simulink model "Two_Zone_MVDC_PSolver_R2020b"  (R2020b)
settings: Solver=FixedStepDiscrete  StartTime=0.0  StopTime=30  FixedStep=TsELEC  RelTol=1e-3  EnableMultiTasking=on
InitFcn:
  | TsELEC = 25e-6;
  | Ts = 25e-6;
  | TsTHERMAL = 1e-3;
  | TsCont = TsELEC;
  | Rsnub = 1e4;
undefined symbols (not defined in the file or in its folder): DiscIntNeverNeededParam, ee_sli_rtmsupport, GABDA, GABDB, GBBDA, GBBDB, gcbh, GPMMA, GPPMB, GPPMC, SADA, SADB, SADC, SADD, SBDA, SBDB, SBDC, SCDA, SCDB, SCDC, SCDD, SDDA, SDDB, SDDC, SDDD, SDDE
libraries: fl_lib x138, nesl_utility x69, ee_lib x52, simulink x3, pid_lib x3, eeTransforms x3, sps_avr x2, powerlib_meascontrol x2, slrealtimetgmanagement x1
(part 2 of 4)

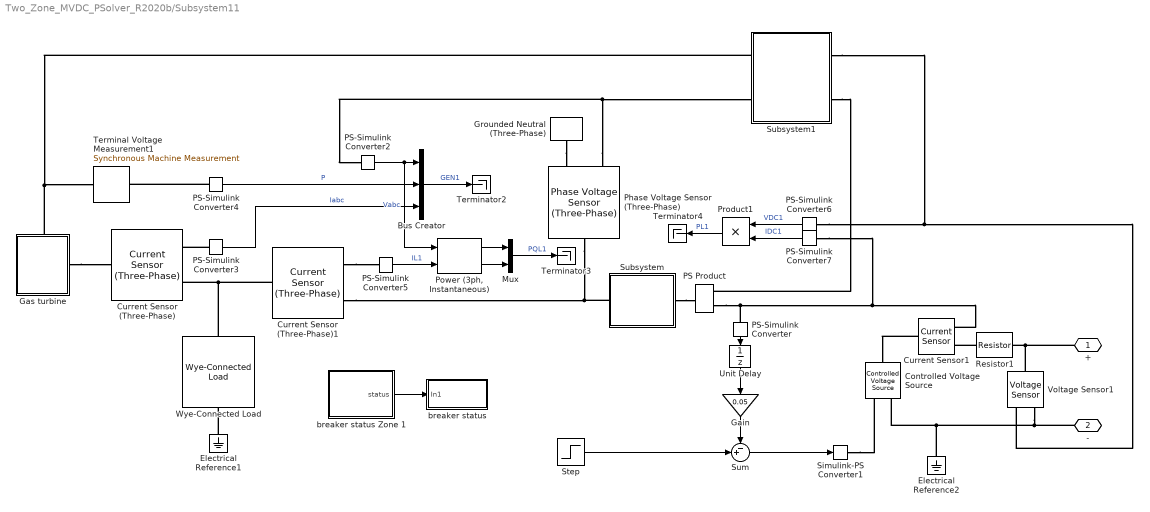
== system Two_Zone_MVDC_PSolver_R2020b/Subsystem11 ==
  Bus Creator : BusCreator  Inputs=3
  Controlled Voltage Source : fl_lib/Electrical/Electrical Sources/Controlled Voltage Source
  Current Sensor (Three-Phase) : ee_lib/Sensors & Transducers/Current Sensor (Three-Phase)
  Current Sensor (Three-Phase)1 : ee_lib/Sensors & Transducers/Current Sensor (Three-Phase)
  Current Sensor1 : fl_lib/Electrical/Electrical Sensors/Current Sensor
  Electrical Reference1 : fl_lib/Electrical/Electrical Elements/Electrical Reference
  Electrical Reference2 : fl_lib/Electrical/Electrical Elements/Electrical Reference
  Gain : Gain  Gain=0.05
  Gas turbine : Subsystem
      settings: PortSchema="{\"entries\":[{\"content\":{\"sides\":[{\"content\":{\"connectorIds\":[]},\"type\":\"ConnectorPlacement.EquallySpacedRectSide\",\"uuid\":\"a1f73c15-13f6-46eb-8342-aad52ebb7cf4\"},{\"content\":{\"connectorIds\":[\"RConn1\"],\"side\":\"RIGHT\"},\"type\":\"ConnectorPlacement.EquallySpacedRectSide\",\"uuid\":\"abeac150-29b8-4860-b513-cf36daae961c\"},{\"content\":{\"connectorIds\":[\"LConn1\"],\"side\":\"TOP\"},\"type\":\"ConnectorPlacement.EquallySpacedRectSide\",\"uuid\":\"5a1fe7e2-6277-4ca3-8dff-8c421d1192c4\"}]},\"type\":\"ConnectorPlacement.EquallySpacedConnector\",\"uuid\":\"d4b4a2cc-ac74-4118-848e-e1a8f51c8633\"}],\"packageUris\":[\"http://schema.mathworks.com/mf0/Connector/19700101\"],\"version\":\"1.0\"}"
  Grounded Neutral (Three-Phase) : ee_lib/Connectors & References/Grounded Neutral (Three-Phase)
      settings: SourceProductBaseCode=PS
  Mux : Mux  Inputs=2
  PS Product : fl_lib/Physical Signals/Functions/PS Product
  PS-Simulink Converter{,2..7} (7 alike) : nesl_utility/PS-Simulink Converter  PhysicalDomain=network_engine_domain  SubClassName=ps_output  LeftPortType=input  RightPortType=output  PseudoPeriodic=off  Frequencies=[]  Unit=inherit  AffineConversion=off
  Phase Voltage Sensor (Three-Phase) : ee_lib/Sensors & Transducers/Phase Voltage Sensor (Three-Phase)
      settings: SourceProductBaseCode=PS
  "Power (3ph, Instantaneous)" : powerlib_meascontrol/Measurements/Power (3ph, Instantaneous)
  Product1 : Product
  Resistor1 : fl_lib/Electrical/Electrical Elements/Resistor  R=1e-5 Ohm  i_specify=off  i_priority=None  i=0 A  i_nominal_specify=off  i_nominal_unit=A  i_nominal_value=1  v_specify=off  v_priority=None  v=0 V  v_nominal_specify=off  v_nominal_unit=V  v_nominal_value=1
  Simulink-PS Converter1 : nesl_utility/Simulink-PS Converter  PhysicalDomain=network_engine_domain  SubClassName=ps_input  LeftPortType=input  RightPortType=output  PseudoPeriodic=off  Frequencies=[]  NoiseDistribution=none  NoiseParameters=[]  Unit=1  AffineConversion=off  FilteringAndDerivatives=provide  SimscapeFilterOrder=1  InputFilterTimeConstant=0.001  UdotUserProvided=0
  Step : Step  Time=12.1  Before=12e3  After=12e3  SampleTime=TsELEC
  Subsystem : Subsystem
  Subsystem1 : Subsystem
  Sum : Sum  Inputs=-+|
  Terminal Voltage Measurement1 : ee_lib/Electromechanical/Synchronous/Synchronous Machine Measurement  output_idx=12
      settings: SourceProductBaseCode=PS  LogSimulationData=on  InternalSimscapePortConfiguration="{\"Bottom\":[],\"Left\":[{\"id\":\"pu_input\",\"label\":\"pu\",\"type\":\"input\"}],\"Right\":[{\"id\":\"pu_output\",\"label\":\"o\",\"type\":\"output\"}],\"Top\":[]}"
  Terminator2 : Terminator
  Terminator3 : Terminator
  Terminator4 : Terminator
  Unit Delay : UnitDelay  SampleTime=TsELEC  HasFrameUpgradeWarning=on
  Voltage Sensor1 : fl_lib/Electrical/Electrical Sensors/Voltage Sensor
  Wye-Connected Load : ee_lib/Passive/RLC Assemblies/Wye-Connected Load  parameterization=2  component_structure=1  component_structure_PQ=1  R=1 Ohm  L=1e-3 H  C=1e-6 F  R_parasitic=1e-6 Ohm  G_parasitic=1e-6 1/Ohm  VRated=13.8e3 V  FRated=60 Hz  P=2.5e6 W  Qpos=1e2 V*A  Qneg=-1e2 V*A  Vmag0=24e3 V  Vang0=0 deg  Freq0=60 Hz  R_parasitic_PQ=1e-6 Ohm  G_parasitic_PQ=1e-6 1/Ohm  IL_specify=on  IL_priority=High  IL=[0, 0, 0] A  IL_nominal_specify=off  IL_nominal_unit=A  IL_nominal_value=1  VC_specify=on  VC_priority=High  VC=[0, 0, 0] V  VC_nominal_specify=off  VC_nominal_unit=V  VC_nominal_value=1
      settings: SourceProductBaseCode=PS
  breaker status : Subsystem
  breaker status Zone 1 : Subsystem
  + : PMIOPort  Side=Right
  - : PMIOPort  Port=2  Side=Right
  wires:
  breaker status Zone 1/1(status) -> breaker status/1(In1)
  Bus Creator/1 -> Terminator2/1  "GEN1"
  PS-Simulink Converter7/1 -> Product1/2  "IDC1"
  "Power (3ph, Instantaneous)"/1 -> Mux/1
  Mux/1 -> Terminator3/1  "PQL1"
  PS-Simulink Converter2/1 -> Bus Creator/1, "Power (3ph, Instantaneous)"/1  "Vabc"
  PS-Simulink Converter5/1 -> "Power (3ph, Instantaneous)"/2  "IL1"
  PS-Simulink Converter4/1 -> Bus Creator/2  "P"
  "Power (3ph, Instantaneous)"/2 -> Mux/2
  Product1/1 -> Terminator4/1  "PL1"
  PS-Simulink Converter6/1 -> Product1/1  "VDC1"
  PS-Simulink Converter3/1 -> Bus Creator/3  "Iabc"
  Step/1 -> Sum/2
  PS-Simulink Converter/1 -> Unit Delay/1
  Sum/1 -> Simulink-PS Converter1/1
  Gain/1 -> Sum/1
  Unit Delay/1 -> Gain/1
  connections:
  Voltage Sensor1/LConn1 -- +/RConn1 -- Resistor1/RConn1
  Subsystem1/RConn1 -- PS-Simulink Converter6/LConn1 -- Voltage Sensor1/RConn1
  Voltage Sensor1/RConn2 -- -/RConn1 -- Electrical Reference2/LConn1 -- Controlled Voltage Source/RConn2
  PS Product/LConn1 -- PS-Simulink Converter7/LConn1 -- Current Sensor1/RConn1 -- PS-Simulink Converter/LConn1
  Phase Voltage Sensor (Three-Phase)/LConn1 -- Current Sensor (Three-Phase)1/RConn2 -- Subsystem/RConn1
  Phase Voltage Sensor (Three-Phase)/RConn1 -- PS-Simulink Converter2/LConn1 -- Subsystem1/LConn2
  Resistor1/LConn1 -- Current Sensor1/RConn2
  Grounded Neutral (Three-Phase)/LConn1 -- Phase Voltage Sensor (Three-Phase)/RConn2
  PS-Simulink Converter3/LConn1 -- Current Sensor (Three-Phase)/RConn1
  Electrical Reference1/LConn1 -- Wye-Connected Load/RConn1
  Current Sensor (Three-Phase)1/LConn1 -- Wye-Connected Load/LConn1 -- Current Sensor (Three-Phase)/RConn2
  Simulink-PS Converter1/RConn1 -- Controlled Voltage Source/RConn1
  Current Sensor (Three-Phase)1/RConn1 -- PS-Simulink Converter5/LConn1
  Current Sensor1/LConn1 -- Controlled Voltage Source/LConn1
  Gas turbine/RConn1 -- Current Sensor (Three-Phase)/LConn1
  PS-Simulink Converter4/LConn1 -- Terminal Voltage Measurement1/RConn1
  Gas turbine/LConn1 -- Subsystem1/LConn1 -- Terminal Voltage Measurement1/LConn1
  Subsystem1/RConn2 -- PS Product/LConn2
  Subsystem/LConn1 -- PS Product/RConn1

== system Two_Zone_MVDC_PSolver_R2020b/Subsystem12 ==
  Inductor2 : fl_lib/Electrical/Electrical Elements/Inductor  l=2.63e-6 H  r=0.16e-3 Ohm  g=0 1/Ohm  i_specify=off  i_priority=None  i=0 A  i_nominal_specify=off  i_nominal_unit=A  i_nominal_value=1  v_specify=off  v_priority=None  v=0 V  v_nominal_specify=off  v_nominal_unit=V  v_nominal_value=1  i_L_specify=off  i_L_priority=High  i_L=0 A  i_L_nominal_specify=off  i_L_nominal_unit=A  i_L_nominal_value=1
  Inductor4 : fl_lib/Electrical/Electrical Elements/Inductor  l=2.63e-6 H  r=0.16e-3 Ohm  g=0 1/Ohm  i_specify=off  i_priority=None  i=0 A  i_nominal_specify=off  i_nominal_unit=A  i_nominal_value=1  v_specify=off  v_priority=None  v=0 V  v_nominal_specify=off  v_nominal_unit=V  v_nominal_value=1  i_L_specify=off  i_L_priority=High  i_L=0 A  i_L_nominal_specify=off  i_L_nominal_unit=A  i_L_nominal_value=1
  Resistor : fl_lib/Electrical/Electrical Elements/Resistor  R=Rsnub Ohm  i_specify=off  i_priority=None  i=0 A  i_nominal_specify=off  i_nominal_unit=A  i_nominal_value=1  v_specify=off  v_priority=None  v=0 V  v_nominal_specify=off  v_nominal_unit=V  v_nominal_value=1
  Resistor1 : fl_lib/Electrical/Electrical Elements/Resistor  R=Rsnub Ohm  i_specify=off  i_priority=None  i=0 A  i_nominal_specify=off  i_nominal_unit=A  i_nominal_value=1  v_specify=off  v_priority=None  v=0 V  v_nominal_specify=off  v_nominal_unit=V  v_nominal_value=1
  "+ " : PMIOPort  Side=Left
  + : PMIOPort  Port=2  Side=Right
  - : PMIOPort  Port=3  Side=Left
  "- " : PMIOPort  Port=4  Side=Right
  connections:
  Inductor2/LConn1 -- "+ "/RConn1 -- Resistor/LConn1
  Inductor4/LConn1 -- -/RConn1 -- Resistor/RConn1
  Inductor2/RConn1 -- Resistor1/LConn1 -- +/RConn1
  Inductor4/RConn1 -- Resistor1/RConn1 -- "- "/RConn1

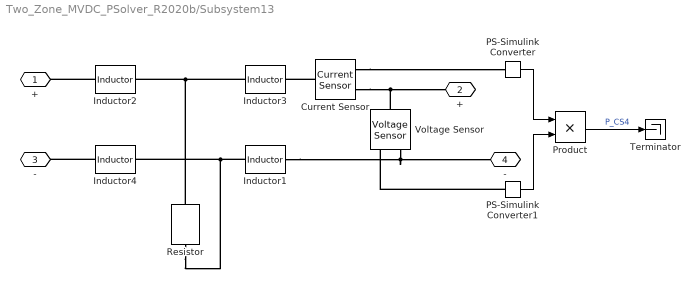
== system Two_Zone_MVDC_PSolver_R2020b/Subsystem13 ==
  Current Sensor : fl_lib/Electrical/Electrical Sensors/Current Sensor
  Inductor{1..4} (4 alike) : fl_lib/Electrical/Electrical Elements/Inductor  l=5e-6/2 H  r=0.2e-3/2 Ohm  g=0 1/Ohm  i_specify=off  i_priority=None  i=0 A  i_nominal_specify=off  i_nominal_unit=A  i_nominal_value=1  v_specify=off  v_priority=None  v=0 V  v_nominal_specify=off  v_nominal_unit=V  v_nominal_value=1  i_L_specify=off  i_L_priority=High  i_L=0 A  i_L_nominal_specify=off  i_L_nominal_unit=A  i_L_nominal_value=1
  PS-Simulink Converter : nesl_utility/PS-Simulink Converter  PhysicalDomain=network_engine_domain  SubClassName=ps_output  LeftPortType=input  RightPortType=output  PseudoPeriodic=off  Frequencies=[]  Unit=inherit  AffineConversion=off
  PS-Simulink Converter1 : nesl_utility/PS-Simulink Converter  PhysicalDomain=network_engine_domain  SubClassName=ps_output  LeftPortType=input  RightPortType=output  PseudoPeriodic=off  Frequencies=[]  Unit=inherit  AffineConversion=off
  Product : Product
  Resistor : fl_lib/Electrical/Electrical Elements/Resistor  R=Rsnub Ohm  i_specify=off  i_priority=None  i=0 A  i_nominal_specify=off  i_nominal_unit=A  i_nominal_value=1  v_specify=off  v_priority=None  v=0 V  v_nominal_specify=off  v_nominal_unit=V  v_nominal_value=1
  Terminator : Terminator
  Voltage Sensor : fl_lib/Electrical/Electrical Sensors/Voltage Sensor
  "+ " : PMIOPort  Side=Left
  + : PMIOPort  Port=2  Side=Right
  - : PMIOPort  Port=3  Side=Left
  "- " : PMIOPort  Port=4  Side=Right
  wires:
  Product/1 -> Terminator/1  "P_CS4"
  PS-Simulink Converter/1 -> Product/1
  PS-Simulink Converter1/1 -> Product/2
  connections:
  Inductor3/LConn1 -- Resistor/LConn1 -- Inductor2/RConn1
  Inductor1/LConn1 -- Resistor/RConn1 -- Inductor4/RConn1
  Current Sensor/LConn1 -- Inductor3/RConn1
  Current Sensor/RConn2 -- Voltage Sensor/LConn1 -- +/RConn1
  Inductor1/RConn1 -- Voltage Sensor/RConn2 -- "- "/RConn1
  Current Sensor/RConn1 -- PS-Simulink Converter/LConn1
  PS-Simulink Converter1/LConn1 -- Voltage Sensor/RConn1
  Inductor2/LConn1 -- "+ "/RConn1
  Inductor4/LConn1 -- -/RConn1

== system Two_Zone_MVDC_PSolver_R2020b/Subsystem14 ==
  Inductor1 : fl_lib/Electrical/Electrical Elements/Inductor  l=5.32e-6 H  r=0.32e-3 Ohm  g=0 1/Ohm  i_specify=off  i_priority=None  i=0 A  i_nominal_specify=off  i_nominal_unit=A  i_nominal_value=1  v_specify=off  v_priority=None  v=0 V  v_nominal_specify=off  v_nominal_unit=V  v_nominal_value=1  i_L_specify=off  i_L_priority=High  i_L=0 A  i_L_nominal_specify=off  i_L_nominal_unit=A  i_L_nominal_value=1
  Inductor2 : fl_lib/Electrical/Electrical Elements/Inductor  l=5.32e-6 H  r=0.32e-3 Ohm  g=0 1/Ohm  i_specify=off  i_priority=None  i=0 A  i_nominal_specify=off  i_nominal_unit=A  i_nominal_value=1  v_specify=off  v_priority=None  v=0 V  v_nominal_specify=off  v_nominal_unit=V  v_nominal_value=1  i_L_specify=off  i_L_priority=High  i_L=0 A  i_L_nominal_specify=off  i_L_nominal_unit=A  i_L_nominal_value=1
  Resistor : fl_lib/Electrical/Electrical Elements/Resistor  R=Rsnub Ohm  i_specify=off  i_priority=None  i=0 A  i_nominal_specify=off  i_nominal_unit=A  i_nominal_value=1  v_specify=off  v_priority=None  v=0 V  v_nominal_specify=off  v_nominal_unit=V  v_nominal_value=1
  "+ " : PMIOPort  Side=Left
  + : PMIOPort  Port=2  Side=Right
  - : PMIOPort  Port=3  Side=Left
  "- " : PMIOPort  Port=4  Side=Right
  connections:
  Inductor1/LConn1 -- Resistor/RConn1 -- -/RConn1
  Inductor2/LConn1 -- Resistor/LConn1 -- "+ "/RConn1
  Inductor2/RConn1 -- +/RConn1
  Inductor1/RConn1 -- "- "/RConn1

== system Two_Zone_MVDC_PSolver_R2020b/Subsystem15 ==
  Inductor1 : fl_lib/Electrical/Electrical Elements/Inductor  l=5.32e-6 H  r=0.32e-3 Ohm  g=0 1/Ohm  i_specify=off  i_priority=None  i=0 A  i_nominal_specify=off  i_nominal_unit=A  i_nominal_value=1  v_specify=off  v_priority=None  v=0 V  v_nominal_specify=off  v_nominal_unit=V  v_nominal_value=1  i_L_specify=off  i_L_priority=High  i_L=0 A  i_L_nominal_specify=off  i_L_nominal_unit=A  i_L_nominal_value=1
  Inductor2 : fl_lib/Electrical/Electrical Elements/Inductor  l=5.32e-6 H  r=0.32e-3 Ohm  g=0 1/Ohm  i_specify=off  i_priority=None  i=0 A  i_nominal_specify=off  i_nominal_unit=A  i_nominal_value=1  v_specify=off  v_priority=None  v=0 V  v_nominal_specify=off  v_nominal_unit=V  v_nominal_value=1  i_L_specify=off  i_L_priority=High  i_L=0 A  i_L_nominal_specify=off  i_L_nominal_unit=A  i_L_nominal_value=1
  Resistor : fl_lib/Electrical/Electrical Elements/Resistor  R=Rsnub Ohm  i_specify=off  i_priority=None  i=0 A  i_nominal_specify=off  i_nominal_unit=A  i_nominal_value=1  v_specify=off  v_priority=None  v=0 V  v_nominal_specify=off  v_nominal_unit=V  v_nominal_value=1
  Resistor1 : fl_lib/Electrical/Electrical Elements/Resistor  R=Rsnub Ohm  i_specify=off  i_priority=None  i=0 A  i_nominal_specify=off  i_nominal_unit=A  i_nominal_value=1  v_specify=off  v_priority=None  v=0 V  v_nominal_specify=off  v_nominal_unit=V  v_nominal_value=1
  "+ " : PMIOPort  Side=Left
  + : PMIOPort  Port=2  Side=Right
  - : PMIOPort  Port=3  Side=Left
  "- " : PMIOPort  Port=4  Side=Right
  connections:
  Inductor1/RConn1 -- Resistor1/LConn1 -- "- "/RConn1
  Inductor2/RConn1 -- Resistor1/RConn1 -- +/RConn1
  Inductor2/LConn1 -- Resistor/LConn1 -- "+ "/RConn1
  Inductor1/LConn1 -- Resistor/RConn1 -- -/RConn1

== system Two_Zone_MVDC_PSolver_R2020b/Subsystem16 ==
  Inductor1 : fl_lib/Electrical/Electrical Elements/Inductor  l=5.32e-6 H  r=0.32e-3 Ohm  g=0 1/Ohm  i_specify=off  i_priority=None  i=0 A  i_nominal_specify=off  i_nominal_unit=A  i_nominal_value=1  v_specify=off  v_priority=None  v=0 V  v_nominal_specify=off  v_nominal_unit=V  v_nominal_value=1  i_L_specify=off  i_L_priority=High  i_L=0 A  i_L_nominal_specify=off  i_L_nominal_unit=A  i_L_nominal_value=1
  Inductor2 : fl_lib/Electrical/Electrical Elements/Inductor  l=5.32e-6 H  r=0.32e-3 Ohm  g=0 1/Ohm  i_specify=off  i_priority=None  i=0 A  i_nominal_specify=off  i_nominal_unit=A  i_nominal_value=1  v_specify=off  v_priority=None  v=0 V  v_nominal_specify=off  v_nominal_unit=V  v_nominal_value=1  i_L_specify=off  i_L_priority=High  i_L=0 A  i_L_nominal_specify=off  i_L_nominal_unit=A  i_L_nominal_value=1
  Resistor : fl_lib/Electrical/Electrical Elements/Resistor  R=Rsnub Ohm  i_specify=off  i_priority=None  i=0 A  i_nominal_specify=off  i_nominal_unit=A  i_nominal_value=1  v_specify=off  v_priority=None  v=0 V  v_nominal_specify=off  v_nominal_unit=V  v_nominal_value=1
  Resistor1 : fl_lib/Electrical/Electrical Elements/Resistor  R=Rsnub Ohm  i_specify=off  i_priority=None  i=0 A  i_nominal_specify=off  i_nominal_unit=A  i_nominal_value=1  v_specify=off  v_priority=None  v=0 V  v_nominal_specify=off  v_nominal_unit=V  v_nominal_value=1
  "+ " : PMIOPort  Side=Left
  + : PMIOPort  Port=2  Side=Right
  - : PMIOPort  Port=3  Side=Left
  "- " : PMIOPort  Port=4  Side=Right
  connections:
  Inductor1/LConn1 -- Resistor/RConn1 -- -/RConn1
  Inductor2/LConn1 -- Resistor/LConn1 -- "+ "/RConn1
  Inductor2/RConn1 -- Resistor1/RConn1 -- +/RConn1
  Inductor1/RConn1 -- Resistor1/LConn1 -- "- "/RConn1

== system Two_Zone_MVDC_PSolver_R2020b/Subsystem2 ==
  Current Sensor : fl_lib/Electrical/Electrical Sensors/Current Sensor
  Inductor1 : fl_lib/Electrical/Electrical Elements/Inductor  l=5e-6 H  r=0.2e-3 Ohm  g=0 1/Ohm  i_specify=off  i_priority=None  i=0 A  i_nominal_specify=off  i_nominal_unit=A  i_nominal_value=1  v_specify=off  v_priority=None  v=0 V  v_nominal_specify=off  v_nominal_unit=V  v_nominal_value=1  i_L_specify=off  i_L_priority=High  i_L=0 A  i_L_nominal_specify=off  i_L_nominal_unit=A  i_L_nominal_value=1
  Inductor3 : fl_lib/Electrical/Electrical Elements/Inductor  l=5e-6 H  r=0.2e-3 Ohm  g=0 1/Ohm  i_specify=off  i_priority=None  i=0 A  i_nominal_specify=off  i_nominal_unit=A  i_nominal_value=1  v_specify=off  v_priority=None  v=0 V  v_nominal_specify=off  v_nominal_unit=V  v_nominal_value=1  i_L_specify=off  i_L_priority=High  i_L=0 A  i_L_nominal_specify=off  i_L_nominal_unit=A  i_L_nominal_value=1
  PS-Simulink Converter : nesl_utility/PS-Simulink Converter  PhysicalDomain=network_engine_domain  SubClassName=ps_output  LeftPortType=input  RightPortType=output  PseudoPeriodic=off  Frequencies=[]  Unit=inherit  AffineConversion=off
  PS-Simulink Converter1 : nesl_utility/PS-Simulink Converter  PhysicalDomain=network_engine_domain  SubClassName=ps_output  LeftPortType=input  RightPortType=output  PseudoPeriodic=off  Frequencies=[]  Unit=inherit  AffineConversion=off
  Product : Product
  Resistor : fl_lib/Electrical/Electrical Elements/Resistor  R=Rsnub Ohm  i_specify=off  i_priority=None  i=0 A  i_nominal_specify=off  i_nominal_unit=A  i_nominal_value=1  v_specify=off  v_priority=None  v=0 V  v_nominal_specify=off  v_nominal_unit=V  v_nominal_value=1
  Resistor1 : fl_lib/Electrical/Electrical Elements/Resistor  R=Rsnub Ohm  i_specify=off  i_priority=None  i=0 A  i_nominal_specify=off  i_nominal_unit=A  i_nominal_value=1  v_specify=off  v_priority=None  v=0 V  v_nominal_specify=off  v_nominal_unit=V  v_nominal_value=1
  Terminator : Terminator
  Voltage Sensor : fl_lib/Electrical/Electrical Sensors/Voltage Sensor
  "+ " : PMIOPort  Side=Left
  + : PMIOPort  Port=2  Side=Right
  - : PMIOPort  Port=3  Side=Left
  "- " : PMIOPort  Port=4  Side=Right
  wires:
  Product/1 -> Terminator/1  "P_CS8"
  PS-Simulink Converter/1 -> Product/1
  PS-Simulink Converter1/1 -> Product/2
  connections:
  Inductor1/LConn1 -- Resistor/RConn1 -- -/RConn1
  Inductor3/LConn1 -- Resistor/LConn1 -- "+ "/RConn1
  Current Sensor/LConn1 -- Resistor1/LConn1 -- Inductor3/RConn1
  Current Sensor/RConn2 -- Voltage Sensor/LConn1 -- +/RConn1
  Inductor1/RConn1 -- Resistor1/RConn1 -- Voltage Sensor/RConn2 -- "- "/RConn1
  Voltage Sensor/RConn1 -- PS-Simulink Converter1/LConn1
  Current Sensor/RConn1 -- PS-Simulink Converter/LConn1

== system Two_Zone_MVDC_PSolver_R2020b/Subsystem3 ==
  Capacitor2 : fl_lib/Electrical/Electrical Elements/Capacitor  c=2e-3 F  r=0 Ohm  g=0 1/Ohm  i_specify=off  i_priority=None  i=0 A  i_nominal_specify=off  i_nominal_unit=A  i_nominal_value=1  v_specify=on  v_priority=None  v=12e3 V  v_nominal_specify=off  v_nominal_unit=V  v_nominal_value=1  vc_specify=on  vc_priority=High  vc=12e3 V  vc_nominal_specify=off  vc_nominal_unit=V  vc_nominal_value=1
  Control : Subsystem
  Current Sensor : fl_lib/Electrical/Electrical Sensors/Current Sensor
  Inverter and PMSM : Subsystem  VariantControl=(sim)
  PS Product : fl_lib/Physical Signals/Functions/PS Product
  PS-Simulink Converter : nesl_utility/PS-Simulink Converter  PhysicalDomain=network_engine_domain  SubClassName=ps_output  LeftPortType=input  RightPortType=output  PseudoPeriodic=off  Frequencies=[]  Unit=inherit  AffineConversion=off
  Speed Reference : Subsystem
  Terminator : Terminator
  Voltage Sensor : fl_lib/Electrical/Electrical Sensors/Voltage Sensor
  + : PMIOPort  Side=Left
  - : PMIOPort  Port=2  Side=Left
  wires:
  PS-Simulink Converter/1 -> Terminator/1  "PDC_motor"
  Control/1(duty_cycle) -> Inverter and PMSM/1(duty_cycle)
  connections:
  PS Product/RConn1 -- PS-Simulink Converter/LConn1
  Voltage Sensor/RConn1 -- PS Product/LConn2
  PS Product/LConn1 -- Current Sensor/RConn1
  Current Sensor/LConn1 -- +/RConn1
  -/RConn1 -- Capacitor2/RConn1 -- Inverter and PMSM/LConn2 -- Voltage Sensor/RConn2
  Capacitor2/LConn1 -- Voltage Sensor/LConn1 -- Current Sensor/RConn2 -- Inverter and PMSM/LConn1

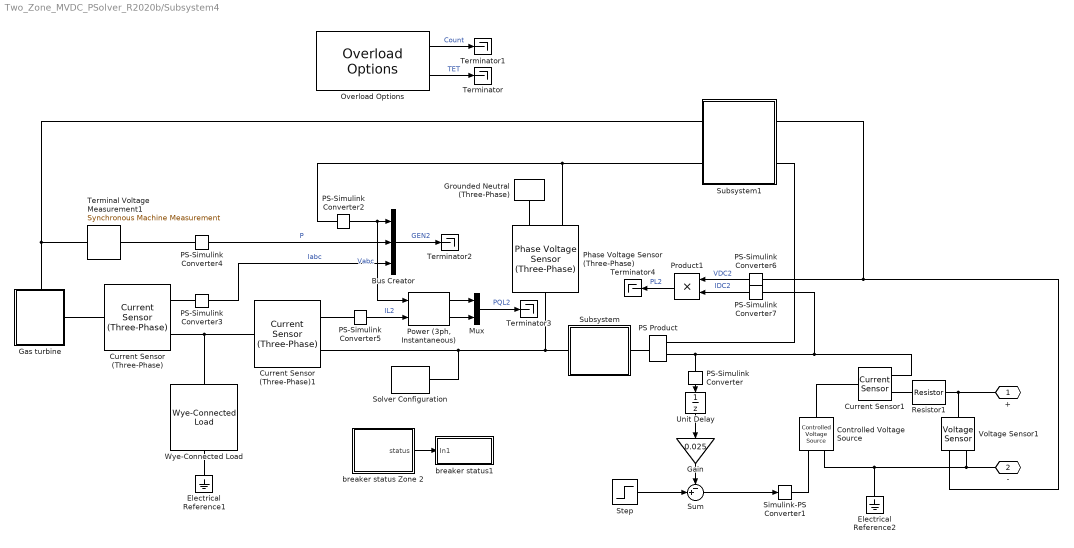
== system Two_Zone_MVDC_PSolver_R2020b/Subsystem4 ==
  Bus Creator : BusCreator  Inputs=3
  Controlled Voltage Source : fl_lib/Electrical/Electrical Sources/Controlled Voltage Source
  Current Sensor (Three-Phase) : ee_lib/Sensors & Transducers/Current Sensor (Three-Phase)
  Current Sensor (Three-Phase)1 : ee_lib/Sensors & Transducers/Current Sensor (Three-Phase)
  Current Sensor1 : fl_lib/Electrical/Electrical Sensors/Current Sensor
  Electrical Reference1 : fl_lib/Electrical/Electrical Elements/Electrical Reference
  Electrical Reference2 : fl_lib/Electrical/Electrical Elements/Electrical Reference
  Gain : Gain  Gain=0.025
  Gas turbine : Subsystem
      settings: PortSchema="{\"entries\":[{\"content\":{\"sides\":[{\"content\":{\"connectorIds\":[]},\"type\":\"ConnectorPlacement.EquallySpacedRectSide\",\"uuid\":\"a1f73c15-13f6-46eb-8342-aad52ebb7cf4\"},{\"content\":{\"connectorIds\":[\"RConn1\"],\"side\":\"RIGHT\"},\"type\":\"ConnectorPlacement.EquallySpacedRectSide\",\"uuid\":\"abeac150-29b8-4860-b513-cf36daae961c\"},{\"content\":{\"connectorIds\":[\"LConn1\"],\"side\":\"TOP\"},\"type\":\"ConnectorPlacement.EquallySpacedRectSide\",\"uuid\":\"5a1fe7e2-6277-4ca3-8dff-8c421d1192c4\"}]},\"type\":\"ConnectorPlacement.EquallySpacedConnector\",\"uuid\":\"d4b4a2cc-ac74-4118-848e-e1a8f51c8633\"}],\"packageUris\":[\"http://schema.mathworks.com/mf0/Connector/19700101\"],\"version\":\"1.0\"}"
  Grounded Neutral (Three-Phase) : ee_lib/Connectors & References/Grounded Neutral (Three-Phase)
      settings: SourceProductBaseCode=PS
  Mux : Mux  Inputs=2
  Overload Options : slrealtimetgmanagement/Overload Options  startupDur=1  startupDurSrc=Tunable Parameter  maxOverload=1000  maxOverloadSrc=Tunable Parameter  TETFlag=on
      settings: SourceProductBaseCode=XP
  PS Product : fl_lib/Physical Signals/Functions/PS Product
  PS-Simulink Converter{,2..7} (7 alike) : nesl_utility/PS-Simulink Converter  PhysicalDomain=network_engine_domain  SubClassName=ps_output  LeftPortType=input  RightPortType=output  PseudoPeriodic=off  Frequencies=[]  Unit=inherit  AffineConversion=off
  Phase Voltage Sensor (Three-Phase) : ee_lib/Sensors & Transducers/Phase Voltage Sensor (Three-Phase)
      settings: SourceProductBaseCode=PS
  "Power (3ph, Instantaneous)" : powerlib_meascontrol/Measurements/Power (3ph, Instantaneous)
  Product1 : Product
  Resistor1 : fl_lib/Electrical/Electrical Elements/Resistor  R=1e-5 Ohm  i_specify=off  i_priority=None  i=0 A  i_nominal_specify=off  i_nominal_unit=A  i_nominal_value=1  v_specify=off  v_priority=None  v=0 V  v_nominal_specify=off  v_nominal_unit=V  v_nominal_value=1
  Simulink-PS Converter1 : nesl_utility/Simulink-PS Converter  PhysicalDomain=network_engine_domain  SubClassName=ps_input  LeftPortType=input  RightPortType=output  PseudoPeriodic=off  Frequencies=[]  NoiseDistribution=none  NoiseParameters=[]  Unit=1  AffineConversion=off  FilteringAndDerivatives=provide  SimscapeFilterOrder=1  InputFilterTimeConstant=0.001  UdotUserProvided=0
  Solver Configuration : nesl_utility/Solver Configuration  PhysicalDomain=network_engine_domain  SubClassName=solver  LeftPortType=input  RightPortType=generic  Tones=[]  Harmonics=[]  SimulateNoise=off  Profile=off  UseLocalSampling=off  EnableSwitchedLinearOptims=on  FrequencyDomain=off  UseCCode=off  RelTol=0.001  AbsTol=1e-06  MinStep=1e-09  ToWorkspace=off  RevertToSquareIcSolve=off  NumHomotopyIterations=100  PhasorMode=off  PhasorModeNumHarmonics=1  DoDC=off  ResidualTolerance=1e-09  UseLocalSolver=on  LocalSolverChoice=NE_PARTITIONING_ADVANCER  LocalSolverSampleTime=TsELEC  DoFixedCost=on  MaxNonlinIter=1  MaxModeIter=2  ComputeImpulses=off  ImpulseIterations=1  LinearAlgebra=auto  EquationFormulation=NE_TIME_EF  DelaysMemoryBudget=1024  AutomaticFiltering=on  FilteringTimeConstant=0.001  PartitionStorageMethod=AS_NEEDED  PartitionMemoryBudget=1024  PartitionMethod=FAST
  Step : Step  Time=12.1  Before=12e3  After=12e3  SampleTime=TsELEC
  Subsystem : Subsystem
  Subsystem1 : Subsystem
  Sum : Sum  Inputs=-+|
  Terminal Voltage Measurement1 : ee_lib/Electromechanical/Synchronous/Synchronous Machine Measurement  output_idx=12
      settings: SourceProductBaseCode=PS  LogSimulationData=on  InternalSimscapePortConfiguration="{\"Bottom\":[],\"Left\":[{\"id\":\"pu_input\",\"label\":\"pu\",\"type\":\"input\"}],\"Right\":[{\"id\":\"pu_output\",\"label\":\"o\",\"type\":\"output\"}],\"Top\":[]}"
  Terminator{,1..4} (5 alike) : Terminator
  Unit Delay : UnitDelay  SampleTime=TsELEC  HasFrameUpgradeWarning=on
  Voltage Sensor1 : fl_lib/Electrical/Electrical Sensors/Voltage Sensor
  Wye-Connected Load : ee_lib/Passive/RLC Assemblies/Wye-Connected Load  parameterization=2  component_structure=1  component_structure_PQ=1  R=1 Ohm  L=1e-3 H  C=1e-6 F  R_parasitic=1e-6 Ohm  G_parasitic=1e-6 1/Ohm  VRated=13.8e3 V  FRated=60 Hz  P=2.5e6 W  Qpos=1e2 V*A  Qneg=-1e2 V*A  Vmag0=24e3 V  Vang0=0 deg  Freq0=60 Hz  R_parasitic_PQ=1e-6 Ohm  G_parasitic_PQ=1e-6 1/Ohm  IL_specify=on  IL_priority=High  IL=[0, 0, 0] A  IL_nominal_specify=off  IL_nominal_unit=A  IL_nominal_value=1  VC_specify=on  VC_priority=High  VC=[0, 0, 0] V  VC_nominal_specify=off  VC_nominal_unit=V  VC_nominal_value=1
      settings: SourceProductBaseCode=PS
  breaker status Zone 2 : Subsystem
  breaker status1 : Subsystem
  + : PMIOPort  Side=Right
  - : PMIOPort  Port=2  Side=Right
  wires:
  breaker status Zone 2/1(status) -> breaker status1/1(In1)
  PS-Simulink Converter6/1 -> Product1/1  "VDC2"
  Product1/1 -> Terminator4/1  "PL2"
  Bus Creator/1 -> Terminator2/1  "GEN2"
  PS-Simulink Converter5/1 -> "Power (3ph, Instantaneous)"/2  "IL2"
  PS-Simulink Converter3/1 -> Bus Creator/3  "Iabc"
  "Power (3ph, Instantaneous)"/1 -> Mux/1
  Mux/1 -> Terminator3/1  "PQL2"
  PS-Simulink Converter2/1 -> Bus Creator/1, "Power (3ph, Instantaneous)"/1  "Vabc"
  PS-Simulink Converter7/1 -> Product1/2  "IDC2"
  "Power (3ph, Instantaneous)"/2 -> Mux/2
  PS-Simulink Converter4/1 -> Bus Creator/2  "P"
  Gain/1 -> Sum/1
  Sum/1 -> Simulink-PS Converter1/1
  Unit Delay/1 -> Gain/1
  Step/1 -> Sum/2
  PS-Simulink Converter/1 -> Unit Delay/1
  Overload Options/2 -> Terminator/1  "TET"
  Overload Options/1 -> Terminator1/1  "Count"
  connections:
  Controlled Voltage Source/RConn2 -- -/RConn1 -- Voltage Sensor1/RConn2 -- Electrical Reference2/LConn1
  Voltage Sensor1/LConn1 -- +/RConn1 -- Resistor1/RConn1
  PS Product/LConn1 -- PS-Simulink Converter/LConn1 -- PS-Simulink Converter7/LConn1 -- Current Sensor1/RConn1
  Phase Voltage Sensor (Three-Phase)/RConn1 -- PS-Simulink Converter2/LConn1 -- Subsystem1/LConn2
  Current Sensor (Three-Phase)1/LConn1 -- Wye-Connected Load/LConn1 -- Current Sensor (Three-Phase)/RConn2
  Subsystem1/RConn1 -- PS-Simulink Converter6/LConn1 -- Voltage Sensor1/RConn1
  Terminal Voltage Measurement1/LConn1 -- Subsystem1/LConn1 -- Gas turbine/LConn1
  Phase Voltage Sensor (Three-Phase)/LConn1 -- Solver Configuration/RConn1 -- Current Sensor (Three-Phase)1/RConn2 -- Subsystem/RConn1
  Current Sensor1/LConn1 -- Controlled Voltage Source/LConn1
  Resistor1/LConn1 -- Current Sensor1/RConn2
  Subsystem1/RConn2 -- PS Product/LConn2
  Simulink-PS Converter1/RConn1 -- Controlled Voltage Source/RConn1
  Electrical Reference1/LConn1 -- Wye-Connected Load/RConn1
  PS-Simulink Converter4/LConn1 -- Terminal Voltage Measurement1/RConn1
  PS-Simulink Converter3/LConn1 -- Current Sensor (Three-Phase)/RConn1
  PS Product/RConn1 -- Subsystem/LConn1
  Gas turbine/RConn1 -- Current Sensor (Three-Phase)/LConn1
  Current Sensor (Three-Phase)1/RConn1 -- PS-Simulink Converter5/LConn1
  Grounded Neutral (Three-Phase)/LConn1 -- Phase Voltage Sensor (Three-Phase)/RConn2

== system Two_Zone_MVDC_PSolver_R2020b/Subsystem5 ==
  Inductor1 : fl_lib/Electrical/Electrical Elements/Inductor  l=5.32e-6 H  r=0.32e-3 Ohm  g=0 1/Ohm  i_specify=off  i_priority=None  i=0 A  i_nominal_specify=off  i_nominal_unit=A  i_nominal_value=1  v_specify=off  v_priority=None  v=0 V  v_nominal_specify=off  v_nominal_unit=V  v_nominal_value=1  i_L_specify=off  i_L_priority=High  i_L=0 A  i_L_nominal_specify=off  i_L_nominal_unit=A  i_L_nominal_value=1
  Inductor2 : fl_lib/Electrical/Electrical Elements/Inductor  l=5.32e-6 H  r=0.32e-3 Ohm  g=0 1/Ohm  i_specify=off  i_priority=None  i=0 A  i_nominal_specify=off  i_nominal_unit=A  i_nominal_value=1  v_specify=off  v_priority=None  v=0 V  v_nominal_specify=off  v_nominal_unit=V  v_nominal_value=1  i_L_specify=off  i_L_priority=High  i_L=0 A  i_L_nominal_specify=off  i_L_nominal_unit=A  i_L_nominal_value=1
  Resistor : fl_lib/Electrical/Electrical Elements/Resistor  R=Rsnub Ohm  i_specify=off  i_priority=None  i=0 A  i_nominal_specify=off  i_nominal_unit=A  i_nominal_value=1  v_specify=off  v_priority=None  v=0 V  v_nominal_specify=off  v_nominal_unit=V  v_nominal_value=1
  Resistor1 : fl_lib/Electrical/Electrical Elements/Resistor  R=Rsnub Ohm  i_specify=off  i_priority=None  i=0 A  i_nominal_specify=off  i_nominal_unit=A  i_nominal_value=1  v_specify=off  v_priority=None  v=0 V  v_nominal_specify=off  v_nominal_unit=V  v_nominal_value=1
  "+ " : PMIOPort  Side=Left
  + : PMIOPort  Port=2  Side=Right
  - : PMIOPort  Port=3  Side=Left
  "- " : PMIOPort  Port=4  Side=Right
  connections:
  Inductor1/RConn1 -- Resistor1/RConn1 -- "- "/RConn1
  Inductor2/RConn1 -- Resistor1/LConn1 -- +/RConn1
  Inductor2/LConn1 -- Resistor/LConn1 -- "+ "/RConn1
  Inductor1/LConn1 -- Resistor/RConn1 -- -/RConn1

== system Two_Zone_MVDC_PSolver_R2020b/Subsystem6 ==
  Inductor1 : fl_lib/Electrical/Electrical Elements/Inductor  l=2.63e-6 H  r=0.16e-3 Ohm  g=0 1/Ohm  i_specify=off  i_priority=None  i=0 A  i_nominal_specify=off  i_nominal_unit=A  i_nominal_value=1  v_specify=off  v_priority=None  v=0 V  v_nominal_specify=off  v_nominal_unit=V  v_nominal_value=1  i_L_specify=off  i_L_priority=High  i_L=0 A  i_L_nominal_specify=off  i_L_nominal_unit=A  i_L_nominal_value=1
  Inductor3 : fl_lib/Electrical/Electrical Elements/Inductor  l=2.63e-6 H  r=0.16e-3 Ohm  g=0 1/Ohm  i_specify=off  i_priority=None  i=0 A  i_nominal_specify=off  i_nominal_unit=A  i_nominal_value=1  v_specify=off  v_priority=None  v=0 V  v_nominal_specify=off  v_nominal_unit=V  v_nominal_value=1  i_L_specify=off  i_L_priority=High  i_L=0 A  i_L_nominal_specify=off  i_L_nominal_unit=A  i_L_nominal_value=1
  Resistor : fl_lib/Electrical/Electrical Elements/Resistor  R=Rsnub Ohm  i_specify=off  i_priority=None  i=0 A  i_nominal_specify=off  i_nominal_unit=A  i_nominal_value=1  v_specify=off  v_priority=None  v=0 V  v_nominal_specify=off  v_nominal_unit=V  v_nominal_value=1
  "+ " : PMIOPort  Side=Left
  + : PMIOPort  Port=2  Side=Right
  - : PMIOPort  Port=3  Side=Left
  "- " : PMIOPort  Port=4  Side=Right
  connections:
  Inductor1/LConn1 -- Resistor/RConn1 -- -/RConn1
  Inductor3/LConn1 -- Resistor/LConn1 -- "+ "/RConn1
  Inductor3/RConn1 -- +/RConn1
  Inductor1/RConn1 -- "- "/RConn1

== system Two_Zone_MVDC_PSolver_R2020b/Subsystem8 ==
  Inductor1 : fl_lib/Electrical/Electrical Elements/Inductor  l=2.63e-6 H  r=0.16e-3 Ohm  g=0 1/Ohm  i_specify=off  i_priority=None  i=0 A  i_nominal_specify=off  i_nominal_unit=A  i_nominal_value=1  v_specify=off  v_priority=None  v=0 V  v_nominal_specify=off  v_nominal_unit=V  v_nominal_value=1  i_L_specify=off  i_L_priority=High  i_L=0 A  i_L_nominal_specify=off  i_L_nominal_unit=A  i_L_nominal_value=1
  Inductor3 : fl_lib/Electrical/Electrical Elements/Inductor  l=2.63e-6 H  r=0.16e-3 Ohm  g=0 1/Ohm  i_specify=off  i_priority=None  i=0 A  i_nominal_specify=off  i_nominal_unit=A  i_nominal_value=1  v_specify=off  v_priority=None  v=0 V  v_nominal_specify=off  v_nominal_unit=V  v_nominal_value=1  i_L_specify=off  i_L_priority=High  i_L=0 A  i_L_nominal_specify=off  i_L_nominal_unit=A  i_L_nominal_value=1
  Resistor : fl_lib/Electrical/Electrical Elements/Resistor  R=Rsnub Ohm  i_specify=off  i_priority=None  i=0 A  i_nominal_specify=off  i_nominal_unit=A  i_nominal_value=1  v_specify=off  v_priority=None  v=0 V  v_nominal_specify=off  v_nominal_unit=V  v_nominal_value=1
  "+ " : PMIOPort  Side=Left
  + : PMIOPort  Port=2  Side=Right
  - : PMIOPort  Port=3  Side=Left
  "- " : PMIOPort  Port=4  Side=Right
  connections:
  Inductor1/RConn1 -- "- "/RConn1
  Inductor3/RConn1 -- +/RConn1
  Inductor3/LConn1 -- Resistor/LConn1 -- "+ "/RConn1
  Inductor1/LConn1 -- Resistor/RConn1 -- -/RConn1

== system Two_Zone_MVDC_PSolver_R2020b/Subsystem9 ==
  Current Sensor : fl_lib/Electrical/Electrical Sensors/Current Sensor
  Inductor1 : fl_lib/Electrical/Electrical Elements/Inductor  l=3.47e-6 H  r=0.21e-3 Ohm  g=0 1/Ohm  i_specify=off  i_priority=None  i=0 A  i_nominal_specify=off  i_nominal_unit=A  i_nominal_value=1  v_specify=off  v_priority=None  v=0 V  v_nominal_specify=off  v_nominal_unit=V  v_nominal_value=1  i_L_specify=off  i_L_priority=High  i_L=0 A  i_L_nominal_specify=off  i_L_nominal_unit=A  i_L_nominal_value=1
  Inductor3 : fl_lib/Electrical/Electrical Elements/Inductor  l=3.47e-6 H  r=0.21e-3 Ohm  g=0 1/Ohm  i_specify=off  i_priority=None  i=0 A  i_nominal_specify=off  i_nominal_unit=A  i_nominal_value=1  v_specify=off  v_priority=None  v=0 V  v_nominal_specify=off  v_nominal_unit=V  v_nominal_value=1  i_L_specify=off  i_L_priority=High  i_L=0 A  i_L_nominal_specify=off  i_L_nominal_unit=A  i_L_nominal_value=1
  PS-Simulink Converter : nesl_utility/PS-Simulink Converter  PhysicalDomain=network_engine_domain  SubClassName=ps_output  LeftPortType=input  RightPortType=output  PseudoPeriodic=off  Frequencies=[]  Unit=inherit  AffineConversion=off
  PS-Simulink Converter1 : nesl_utility/PS-Simulink Converter  PhysicalDomain=network_engine_domain  SubClassName=ps_output  LeftPortType=input  RightPortType=output  PseudoPeriodic=off  Frequencies=[]  Unit=inherit  AffineConversion=off
  Product : Product
  Resistor : fl_lib/Electrical/Electrical Elements/Resistor  R=Rsnub Ohm  i_specify=off  i_priority=None  i=0 A  i_nominal_specify=off  i_nominal_unit=A  i_nominal_value=1  v_specify=off  v_priority=None  v=0 V  v_nominal_specify=off  v_nominal_unit=V  v_nominal_value=1
  Terminator : Terminator
  Voltage Sensor : fl_lib/Electrical/Electrical Sensors/Voltage Sensor
  "+ " : PMIOPort  Side=Left
  + : PMIOPort  Port=2  Side=Right
  - : PMIOPort  Port=3  Side=Left
  "- " : PMIOPort  Port=4  Side=Right
  wires:
  PS-Simulink Converter/1 -> Product/1
  PS-Simulink Converter1/1 -> Product/2
  Product/1 -> Terminator/1  "P_CS2"
  connections:
  Inductor3/LConn1 -- "+ "/RConn1
  Inductor1/LConn1 -- -/RConn1
  Inductor1/RConn1 -- Resistor/RConn1 -- Voltage Sensor/RConn2 -- "- "/RConn1
  Current Sensor/LConn1 -- Resistor/LConn1 -- Inductor3/RConn1
  Current Sensor/RConn2 -- Voltage Sensor/LConn1 -- +/RConn1
  PS-Simulink Converter/LConn1 -- Current Sensor/RConn1
  PS-Simulink Converter1/LConn1 -- Voltage Sensor/RConn1

== system Two_Zone_MVDC_PSolver_R2020b/Subsystem11/Gas turbine ==
  " AVR and exciter" : Subsystem
  Electrical Reference : fl_lib/Electrical/Electrical Elements/Electrical Reference
  Inertia : ee_lib/Electromechanical/Mechanical/Machine Inertia  SRated=36e6 V*A  FRated=60 Hz  nPolePairs=1  inertia_option=2  J=27548 kg*m^2  H=2.525 s*W/V/A  damper_option=2  D=39.0509 N*m/(rad/s)  pu_D=0.01  initialization_option=2  fMechanical0=60 Hz  fElectrical0=60 Hz
      settings: SourceProductBaseCode=PS  LogSimulationData=on  InternalSimscapePortConfiguration="{\"Bottom\":[],\"Left\":[{\"id\":\"R\",\"label\":\"R\",\"type\":\"foundation.mechanical.rotational.rotational\"}],\"Right\":[],\"Top\":[]}"
  Synchronous Machine Salient Pole : ee_lib/Electromechanical/Synchronous/Synchronous Machine Salient Pole  SRated=36e6 V*A  VRated=13.8e3 V  FRated=60 Hz  nPolePairs=1  param_option=ee.enum.sm.parameterization.standard  fieldCircuitParameterization_option=ee.enum.sm.fieldparameterization.current  baseEfd=216.54 V  baseIfd=200 A  zero_sequence=ee.enum.park.zerosequence.exclude  Ladu=0.9  Laqu=0.55  L0=0.15  Ll=0.15  Ra=0.006  Lfd=0.2571  Rfd=0.0006  L1d=0.2  R1d=0.0354  L1q=0.2567  R1q=0.0428  Xl=0.08  Xd=1.352  Xq=0.836  X0=0.15  Xdd=0.296  Xddd=0.148  Xqdd=0.122  d_option=ee.enum.circuit.open  Td0d=4.141 s  Tdd=1.75 s  Td0dd=0.027 s  Tddd=0.0214 s  q_option=ee.enum.circuit.open  Tq0dd=0.184 s  Tqdd=0.0232 s  saturation_option=ee.enum.saturation.exclude  axes_param=ee.enum.rotorangle.daxis  saturation_ifd=[0, .48, .76, 1.38, 1.79]  saturation_Vag=[0, .43, .59, .71, .76]  initialization_option=ee.enum.sm.initialization.electrical  source_type=ee.enum.sm.load_flow_source_type.Swing  Vmag0=13.8e3 V  Vang0=0 deg  Pt0=2e6 V*A  Qt0=0 V*A  minimum_pu=0.95  phase_search_range=[-30, 30] deg  gmin=1e-6 S  connection_option=ee.enum.Connection.wye  num_q_dampers=1  rotor_offset=-pi / 2 rad  pu_psid_specify=off  pu_psid_priority=None  pu_psid=0  pu_psid_nominal_specify=off  pu_psid_nominal_unit=1  pu_psid_nominal_value=1  pu_psiq_specify=off  pu_psiq_priority=None  pu_psiq=0  pu_psiq_nominal_specify=off  pu_psiq_nominal_unit=1  pu_psiq_nominal_value=1  pu_psifd_specify=off  pu_psifd_priority=None  pu_psifd=0  pu_psifd_nominal_specify=off  pu_psifd_nominal_unit=1  pu_psifd_nominal_value=1  pu_psi1d_specify=off  pu_psi1d_priority=None  pu_psi1d=0  pu_psi1d_nominal_specify=off  pu_psi1d_nominal_unit=1  pu_psi1d_nominal_value=1  pu_psi1q_specify=off  pu_psi1q_priority=None  pu_psi1q=0  pu_psi1q_nominal_specify=off  pu_psi1q_nominal_unit=1  pu_psi1q_nominal_value=1  angular_position_diff_specify=off  angular_position_diff_priority=None  angular_position_diff=18 deg  angular_position_diff_nominal_specify=off  angular_position_diff_nominal_unit=deg  angular_position_diff_nominal_value=1
      settings: SourceProductBaseCode=PS  InternalSimscapePortConfiguration="{\"Bottom\":[],\"Left\":[{\"id\":\"fd_p\",\"label\":\"fd+\",\"type\":\"foundation.electrical.electrical\"},{\"id\":\"fd_n\",\"label\":\"fd-\",\"type\":\"foundation.electrical.electrical\"},{\"id\":\"R\",\"label\":\"R\",\"type\":\"foundation.mechanical.rotational.rotational\"},{\"id\":\"C\",\"label\":\"C\",\"type\":\"foundation.mechanical.rotational.rotational\"}],\"Right\":[{\"id\":\"pu_output\",\"label\":\"pu\",\"type\":\"output\"},{\"id\":\"N\",\"label\":\"~\",\"type\":\"foundation.electrical.three_phase\"},{\"id\":\"n\",\"label\":\"n\",\"type\":\"foundation.electrical.electrical\"}],\"Top\":[]}"
  "Turbine and governor " : Subsystem  mask(Governor and Prime Mover){pu_speed_reference=0.998, droop_percentage=5, pu_load_reference_setpoint=0.5, T_G=0.1, T_GT=0.2, base_torque=79577.5, pu_torque0=0.500751}
      mask prompts: pu_speed_reference "Speed reference, (pu)"; droop_percentage "Percentage droop, (%)"; pu_load_reference_setpoint "Load reference setpoint, (pu)"; T_G "Time constant of governor, (s)"; T_GT "Time constant of gas turbine, (s)"; base_torque "Base torque, (N*m)"; pu_torque0 "Initial torque, (pu)"
      mask help:
      | Implements a synchronous machine governor and prime mover. The prime mover is a gas turbine.
      |
      | The input to the block is a per-unit synchronous machine measurement vector.
      |
      | R and C are mechanical rotational ports.
  meas : PMIOPort  Side=Left
  ~ : PMIOPort  Port=2  Side=Right
  connections:
  " AVR and exciter"/RConn1 -- Synchronous Machine Salient Pole/LConn1
  Synchronous Machine Salient Pole/LConn4 -- "Turbine and governor "/RConn2
  "Turbine and governor "/LConn1 -- " AVR and exciter"/LConn1 -- Synchronous Machine Salient Pole/RConn1 -- meas/RConn1
  Inertia/LConn1 -- "Turbine and governor "/RConn1 -- Synchronous Machine Salient Pole/LConn3
  " AVR and exciter"/RConn2 -- Synchronous Machine Salient Pole/LConn2
  Synchronous Machine Salient Pole/RConn3 -- Electrical Reference/LConn1
  Synchronous Machine Salient Pole/RConn2 -- ~/RConn1

== system Two_Zone_MVDC_PSolver_R2020b/Subsystem11/Subsystem ==
  Controlled Current Source : fl_lib/Electrical/Electrical Sources/Controlled Current Source
  Controlled Current Source1 : fl_lib/Electrical/Electrical Sources/Controlled Current Source
  Controlled Current Source2 : fl_lib/Electrical/Electrical Sources/Controlled Current Source
  Electrical Reference2 : fl_lib/Electrical/Electrical Elements/Electrical Reference
  Phase Splitter : ee_lib/Connectors & References/Phase Splitter
      settings: SourceProductBaseCode=PS
  Three Element Demux : ee_lib/Connectors & References/Three Element Demux
      settings: SourceProductBaseCode=PS  InternalSimscapePortConfiguration="{\"Bottom\":[],\"Left\":[{\"id\":\"abc\",\"label\":\"abc\",\"type\":\"input\"}],\"Right\":[{\"id\":\"a\",\"label\":\"a\",\"type\":\"output\"},{\"id\":\"b\",\"label\":\"b\",\"type\":\"output\"},{\"id\":\"c\",\"label\":\"c\",\"type\":\"output\"}],\"Top\":[]}"
  ~ : PMIOPort  Side=Right
  mod : PMIOPort  Port=2  Side=Left
  connections:
  Three Element Demux/LConn1 -- mod/RConn1
  Three Element Demux/RConn1 -- Controlled Current Source/RConn1
  Three Element Demux/RConn2 -- Controlled Current Source1/RConn1
  Controlled Current Source2/RConn1 -- Three Element Demux/RConn3
  Phase Splitter/RConn3 -- Controlled Current Source2/LConn1
  ~/RConn1 -- Phase Splitter/LConn1
  Phase Splitter/RConn2 -- Controlled Current Source1/LConn1
  Phase Splitter/RConn1 -- Controlled Current Source/LConn1
  Controlled Current Source2/RConn2 -- Controlled Current Source1/RConn2 -- Controlled Current Source/RConn2 -- Electrical Reference2/LConn1

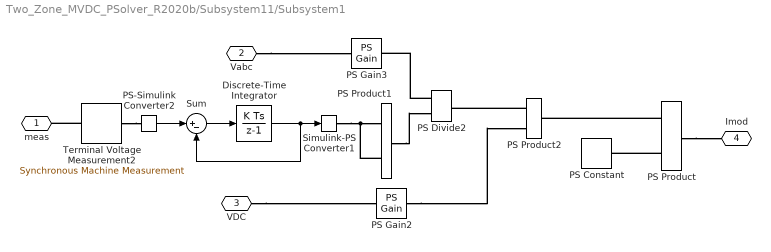
== system Two_Zone_MVDC_PSolver_R2020b/Subsystem11/Subsystem1 ==
  Discrete-Time Integrator : DiscreteIntegrator  gainval=200  InitialCondition=1  SampleTime=TsELEC  ICPrevOutput=DiscIntNeverNeededParam  ICPrevScaledInput=DiscIntNeverNeededParam
  PS Constant : fl_lib/Physical Signals/Sources/PS Constant  constant=-12/13.8 1/V/A
  PS Divide2 : fl_lib/Physical Signals/Functions/PS Divide
      settings: SourceProductBaseCode=SS
  PS Gain2 : fl_lib/Physical Signals/Functions/PS Gain  gain=1/12e3 1/V
  PS Gain3 : fl_lib/Physical Signals/Functions/PS Gain  gain=1/13.8e3
  PS Product : fl_lib/Physical Signals/Functions/PS Product
  PS Product1 : fl_lib/Physical Signals/Functions/PS Product
  PS Product2 : fl_lib/Physical Signals/Functions/PS Product
  PS-Simulink Converter2 : nesl_utility/PS-Simulink Converter  PhysicalDomain=network_engine_domain  SubClassName=ps_output  LeftPortType=input  RightPortType=output  PseudoPeriodic=off  Frequencies=[]  Unit=inherit  AffineConversion=off
  Simulink-PS Converter1 : nesl_utility/Simulink-PS Converter  PhysicalDomain=network_engine_domain  SubClassName=ps_input  LeftPortType=input  RightPortType=output  PseudoPeriodic=off  Frequencies=[]  NoiseDistribution=none  NoiseParameters=[]  Unit=1  AffineConversion=off  FilteringAndDerivatives=provide  SimscapeFilterOrder=1  InputFilterTimeConstant=0.001  UdotUserProvided=0
  Sum : Sum  Inputs=|+-
  Terminal Voltage Measurement2 : ee_lib/Electromechanical/Synchronous/Synchronous Machine Measurement  output_idx=14
      settings: SourceProductBaseCode=PS  LogSimulationData=on  InternalSimscapePortConfiguration="{\"Bottom\":[],\"Left\":[{\"id\":\"pu_input\",\"label\":\"pu\",\"type\":\"input\"}],\"Right\":[{\"id\":\"pu_output\",\"label\":\"o\",\"type\":\"output\"}],\"Top\":[]}"
  meas : PMIOPort  Side=Left
  Vabc : PMIOPort  Port=2  Side=Left
  VDC : PMIOPort  Port=3  Side=Right
  Imod : PMIOPort  Port=4  Side=Right
  wires:
  Sum/1 -> Discrete-Time Integrator/1
  Discrete-Time Integrator/1 -> Sum/2, Simulink-PS Converter1/1
  PS-Simulink Converter2/1 -> Sum/1
  connections:
  PS Product1/RConn1 -- PS Divide2/LConn2
  PS Product/LConn1 -- PS Product2/RConn1
  Vabc/RConn1 -- PS Gain3/LConn1
  PS Gain2/RConn1 -- PS Product2/LConn2
  PS Product/RConn1 -- Imod/RConn1
  VDC/RConn1 -- PS Gain2/LConn1
  PS Product2/LConn1 -- PS Divide2/RConn1
  PS Product/LConn2 -- PS Constant/RConn1
  Terminal Voltage Measurement2/LConn1 -- meas/RConn1
  PS Divide2/LConn1 -- PS Gain3/RConn1
  Terminal Voltage Measurement2/RConn1 -- PS-Simulink Converter2/LConn1
  Simulink-PS Converter1/RConn1 -- PS Product1/LConn2 -- PS Product1/LConn1

== system Two_Zone_MVDC_PSolver_R2020b/Subsystem11/breaker status ==
  In1 : Inport
  Demux : Demux  Outputs=[5 4]
  Demux1 : Demux
  Demux2 : Demux  Outputs=5
  tag scope: GABDA=global, GABDB=global, SADA=global, SADB=global, SADC=global, SADD=global, SBDA=global, SBDB=global, SBDC=global
  wires:
  Demux1/4 -> [GABDB]
  Demux1/3 -> [SBDC]
  Demux1/2 -> [SBDB]
  Demux1/1 -> [SBDA]
  Demux/2 -> Demux1/1
  Demux/1 -> Demux2/1
  In1/1 -> Demux/1
  Demux2/4 -> [SADD]
  Demux2/3 -> [SADC]
  Demux2/1 -> [SADA]
  Demux2/2 -> [SADB]
  Demux2/5 -> [GABDA]

== system Two_Zone_MVDC_PSolver_R2020b/Subsystem11/breaker status Zone 1 ==
  Constant1 : Constant  Value=SBDA  SampleTime=Ts
  Constant2 : Constant  Value=SADA  SampleTime=Ts
  Constant3 : Constant  Value=SADB  SampleTime=Ts
  Constant4 : Constant  Value=SADC  SampleTime=Ts
  Constant5 : Constant  Value=SADD  SampleTime=Ts
  Constant6 : Constant  Value=GABDA  SampleTime=Ts
  Constant7 : Constant  Value=SBDB  SampleTime=Ts
  Constant8 : Constant  Value=SBDC  SampleTime=Ts
  Constant9 : Constant  Value=GABDB  SampleTime=Ts
  Mux : Mux  Inputs=[5 4]
  Mux1 : Mux  Inputs=5
  Mux2 : Mux
  status : Outport  VectorParamsAs1DForOutWhenUnconnected=off
  wires:
  Constant5/1 -> Mux1/4  "SADD"
  Constant2/1 -> Mux1/1  "SADA"
  Constant3/1 -> Mux1/2  "SADB"
  Constant4/1 -> Mux1/3  "SADC"
  Constant6/1 -> Mux1/5  "GABDA"
  Constant1/1 -> Mux2/1  "SBDA"
  Constant7/1 -> Mux2/2  "SBDB"
  Constant8/1 -> Mux2/3  "SBDC"
  Constant9/1 -> Mux2/4  "GABDB"
  Mux/1 -> status/1
  Mux1/1 -> Mux/1
  Mux2/1 -> Mux/2

== system Two_Zone_MVDC_PSolver_R2020b/Subsystem3/Control ==
  Selector : Selector  InputPortWidth=2  IndexOptions=Index vector (dialog)  Indices=2  OutputSizes=1
  Selector1 : Selector  InputPortWidth=2  IndexOptions=Index vector (dialog)  Indices=1  OutputSizes=1
  Speed Control : Subsystem
  Torque Control : Subsystem
  Unit Delay1 : UnitDelay  SampleTime=Ts  HasFrameUpgradeWarning=on
  duty_cycle : Outport
  wires:
  Unit Delay1/1 -> duty_cycle/1
  [Nref1] -> Speed Control/1(Speed_Ref_PU)
  [pos_speed_1] -> Selector/1, Selector1/1
  Selector/1 -> Speed Control/2(Speed_Meas_PU)
  [Iab_meas1] -> Torque Control/2(Iab_Sim)
  Torque Control/1(Vabc_out_PU) -> Unit Delay1/1
  Selector1/1 -> Torque Control/3(Pos_Sim)
  Speed Control/1(IdqRef_PU) -> Torque Control/1(Idq_ref_PU)
